simulink model "fitros"  (R2023b)
settings: Solver=VariableStepAuto  StartTime=0.0  StopTime=100  RelTol=1e-3
settings Model: Creator=mluser  LastModifiedBy=mluser
settings ModelReferenceCC: EnableRefExpFcnMdlSchedulingChecks=on

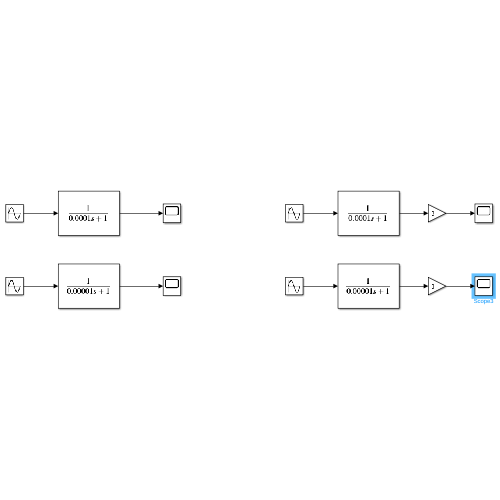
[thumbnail: Simulink's stored preview of the top-level diagram]
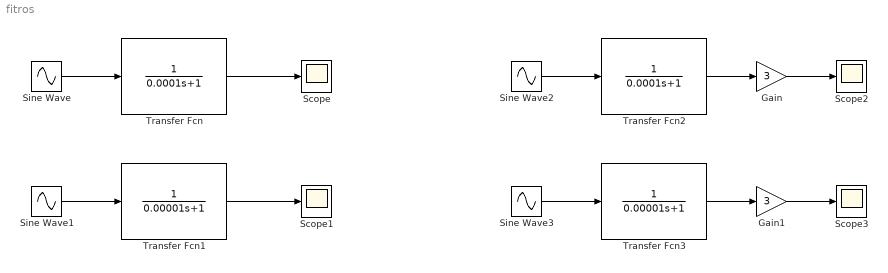
== system fitros ==
  Gain : Gain  Gain=3
  Gain1 : Gain  Gain=3
  Scope{,1..3} (4 alike) : Scope
  Sine Wave : Sin  Amplitude=5  Frequency=6283.1853071796  SampleTime=0
  Sine Wave1 : Sin  Amplitude=5  Frequency=6283.1853071796  SampleTime=0
  Sine Wave2 : Sin  Amplitude=27  Frequency=6283.1853071796  SampleTime=0
  Sine Wave3 : Sin  Amplitude=27  Frequency=6283.1853071796  SampleTime=0
  Transfer Fcn : TransferFcn  Denominator=[0.0001 1]
  Transfer Fcn1 : TransferFcn  Denominator=[0.00001 1]
  Transfer Fcn2 : TransferFcn  Denominator=[0.0001 1]
  Transfer Fcn3 : TransferFcn  Denominator=[0.00001 1]
  wires:
  Sine Wave/1 -> Transfer Fcn/1
  Transfer Fcn/1 -> Scope/1
  Sine Wave1/1 -> Transfer Fcn1/1
  Transfer Fcn1/1 -> Scope1/1
  Sine Wave2/1 -> Transfer Fcn2/1
  Sine Wave3/1 -> Transfer Fcn3/1
  Transfer Fcn2/1 -> Gain/1
  Gain/1 -> Scope2/1
  Gain1/1 -> Scope3/1
  Transfer Fcn3/1 -> Gain1/1
